simulink subsystem "PID_"  (R2020b)
settings: Solver=VariableStepAuto  StartTime=0.0  StopTime=10.0  RelTol=1e-3
model mask{Kp=1.8, Ki=0.075, Kc=0.9, High=60, Low=0}
  mask prompts: Kp "Prop"; Ki "Int"; Kc "Sat"; High "Lim High"; Low "Lim Low"
libraries: simulink x1
settings Model: Creator=a.ermakov  LastModifiedBy=a.ermakov

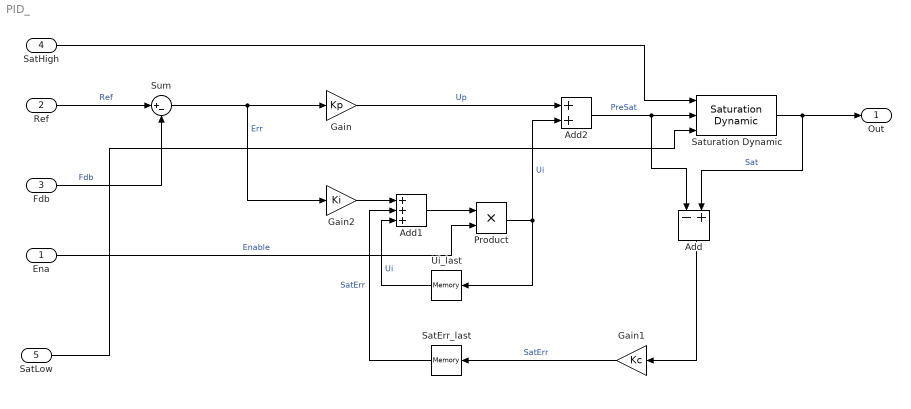
== system PID_ ==
  Ena : Inport
  Ref : Inport  Port=2
  Fdb : Inport  Port=3
  SatHigh : Inport  Port=4
  SatLow : Inport  Port=5
  Add : Sum  Inputs=-+
  Add1 : Sum  Inputs=+++
  Add2 : Sum
  Gain : Gain  Gain=Kp
  Gain1 : Gain  Gain=Kc
  Gain2 : Gain  Gain=Ki
  Product : Product  OutDataTypeStr=single
  SatErr_last : Memory  InheritSampleTime=on
  Saturation Dynamic : simulink/Discontinuities/Saturation Dynamic  OutMin=[]  OutMax=[]  OutDataTypeStr=Inherit: Same as second input  OutDataType=fixdt(1, 16)  OutScaling=2^-10  DoSatur=off
  Sum : Sum  Inputs=|+-
  Ui_last : Memory  InheritSampleTime=on
  Out : Outport
  wires:
  Ena/1 -> Product/2  "Enable"
  Add1/1 -> Product/1
  SatErr_last/1 -> Add1/2  "SatErr"
  Gain/1 -> Add2/1  "Up"
  Ui_last/1 -> Add1/3  "Ui"
  Gain1/1 -> SatErr_last/1  "SatErr"
  Product/1 -> Ui_last/1, Add2/2  "Ui"
  Gain2/1 -> Add1/1
  Sum/1 -> Gain2/1, Gain/1  "Err"
  Fdb/1 -> Sum/2  "Fdb"
  Ref/1 -> Sum/1  "Ref"
  Add/1 -> Gain1/1
  Saturation Dynamic/1 -> Out/1, Add/2  "Sat"
  Add2/1 -> Saturation Dynamic/2, Add/1  "PreSat"
  SatHigh/1 -> Saturation Dynamic/1
  SatLow/1 -> Saturation Dynamic/3
